simulink model "Projekt_FARE2_SS19_template_lyu"  (R2019a)
settings: Solver=ode4  StartTime=0  StopTime=5  FixedStep=0.001  MaxStep=0.001  MinStep=1e-6  RelTol=1e-3  AbsTol=1e-3
PostLoadFcn:
  | %plot(Pos_x(:,2),Pos_y(:,2));
  | %xlabel('x(m)');
  | %ylabel('y(m)');
StopFcn:
  | plot(Pos_x(:,2),Pos_y(:,2));
  | xlabel('x(m)');
  | ylabel('y(m)');
undefined symbols (not defined in the file or in its folder): in
settings Model: Creator=vivgove  LastModifiedBy=eason
settings SolverCC: AutoScaleAbsTol=off  InitialStep=0.001  MaxOrder=3  AutoInsertRateTranBlk=on  InsertRTBMode=Never (minimum delay)
settings DataIOCC: SaveFormat=Array  SignalLoggingSaveFormat=ModelDataLogs  SaveOutput=off  SignalLogging=off  SaveTime=off  ReturnWorkspaceOutputs=off  OutputOption=SpecifiedOutputTimes  OutputTimes=[time]
settings OptimizationCC: DefaultParameterBehavior=Inlined  ExpressionDepthLimit=2147483647  EfficientMapNaN2IntZero=off  LifeSpan=inf
settings DebuggingCC: UnderspecifiedInitializationDetection=Classic  MergeDetectMultiDrivingBlocksExec=none  SolverPrmCheckMsg=warning  FcnCallInpInsideContextMsg=warning  AllowSymbolicDim=off  StateNameClashWarn=warning  SFUnexpectedBacktrackingDiag=warning  SFNoUnconditionalDefaultTransitionDiag=warning  SFExecutionAtInitializationDiag=none  ArithmeticOperatorsInVariantConditions=warning
settings HardwareCC: ProdBitPerPointer=32  ProdBitPerSizeT=32  ProdBitPerPtrDiffT=32  ProdLargestAtomicFloat=None  ProdIntDivRoundTo=Undefined  ProdEndianess=Unspecified  ProdWordSize=32  ProdHWDeviceType=32-bit Generic  TargetBitPerLong=64  TargetBitPerPointer=64  TargetBitPerSizeT=64  TargetBitPerPtrDiffT=64  TargetLongLongMode=on  TargetIntDivRoundTo=Zero  TargetEndianess=LittleEndian  TargetWordSize=64  TargetHWDeviceType=MATLAB Host  ProdEqTarget=off
settings ModelReferenceCC: PropagateSignalLabelsOutOfModel=off
settings SFSimCC: SimUseLocalCustomCode=off
settings RTWCC: RTWUseLocalCustomCode=off
settings CodeAppCC: MaxIdLength=128  StateflowObjectComments=on
settings GRTTargetCC: TargetLangStandard=C89/C90 (ANSI)  CombineOutputUpdateFcns=off  GRTInterface=on
settings ConfigComp: CovMetricSettings=dw  CovHtmlReporting=on  CovSaveCumulativeToWorkspaceVar=on  CovSaveSingleToWorkspaceVar=on  CovExternalEMLEnable=off

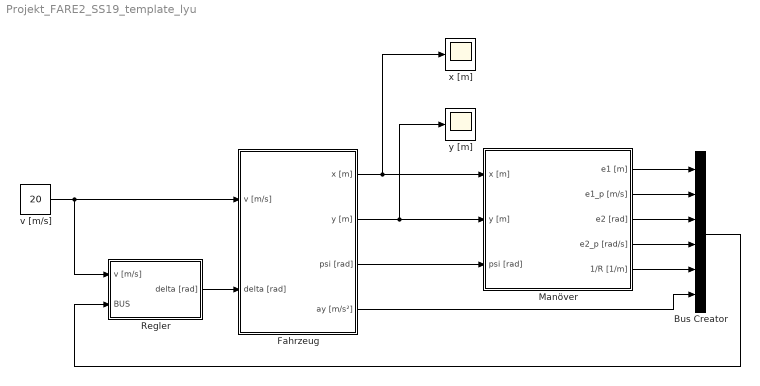
== system Projekt_FARE2_SS19_template_lyu ==
  Bus Creator : BusCreator  Inputs=6
  Fahrzeug : Subsystem
  Manöver : Subsystem
  Regler : Subsystem
  v [m/s] : Constant  Value=20
  x [m] : Scope
  y [m] : Scope
  wires:
  Manöver/1(e1 [m]) -> Bus Creator/1
  Manöver/2(e1_p [m/s]) -> Bus Creator/2
  Manöver/3(e2 [rad]) -> Bus Creator/3
  Manöver/4(e2_p [rad/s]) -> Bus Creator/4
  Manöver/5(1/R [1/m]) -> Bus Creator/5
  Bus Creator/1 -> Regler/2(BUS)
  Fahrzeug/1(x [m]) -> Manöver/1(x [m]), x [m]/1
  Fahrzeug/2(y [m]) -> Manöver/2(y [m]), y [m]/1
  Regler/1(delta [rad]) -> Fahrzeug/2(delta [rad])
  Fahrzeug/3(psi [rad]) -> Manöver/3(psi [rad])
  Fahrzeug/4(ay [m/s²]) -> Bus Creator/6
  v [m/s]/1 -> Regler/1(v [m/s]), Fahrzeug/1(v [m/s])

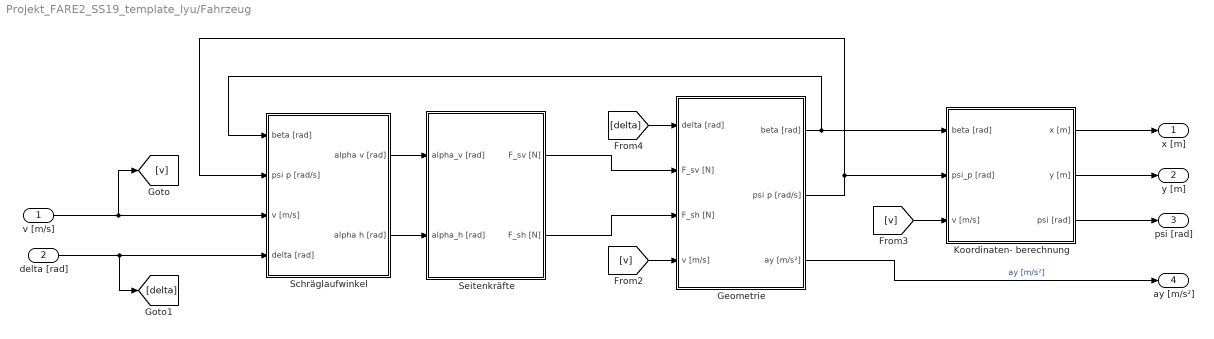
== system Projekt_FARE2_SS19_template_lyu/Fahrzeug ==
  v [m/s] : Inport
  delta [rad] : Inport  Port=2
  Geometrie : Subsystem
  Koordinaten- berechnung : Subsystem
  Schräglaufwinkel : Subsystem
  Seitenkräfte : Subsystem
  x [m] : Outport
  y [m] : Outport  Port=2
  psi [rad] : Outport  Port=3
  ay [m/s²] : Outport  Port=4
  wires:
  [v] -> Koordinaten- berechnung/3(v [m/s])
  [v] -> Geometrie/4(v [m/s])
  [delta] -> Geometrie/1(delta [rad])
  v [m/s]/1 -> Schräglaufwinkel/3(v [m/s]), [v]
  Seitenkräfte/2(F_sh [N]) -> Geometrie/3(F_sh [N])
  Koordinaten- berechnung/3(psi [rad]) -> psi [rad]/1
  Koordinaten- berechnung/1(x [m]) -> x [m]/1
  Geometrie/2(psi p [rad/s]) -> Schräglaufwinkel/2(psi p [rad/s]), Koordinaten- berechnung/2(psi_p [rad])
  Schräglaufwinkel/2(alpha h [rad]) -> Seitenkräfte/2(alpha_h [rad])
  Koordinaten- berechnung/2(y [m]) -> y [m]/1
  Seitenkräfte/1(F_sv [N]) -> Geometrie/2(F_sv [N])
  Geometrie/1(beta [rad]) -> Koordinaten- berechnung/1(beta [rad]), Schräglaufwinkel/1(beta [rad])
  Schräglaufwinkel/1(alpha v [rad]) -> Seitenkräfte/1(alpha_v [rad])
  Geometrie/3(ay [m/s²]) -> ay [m/s²]/1  "ay [m/s²]"
  delta [rad]/1 -> [delta], Schräglaufwinkel/4(delta [rad])

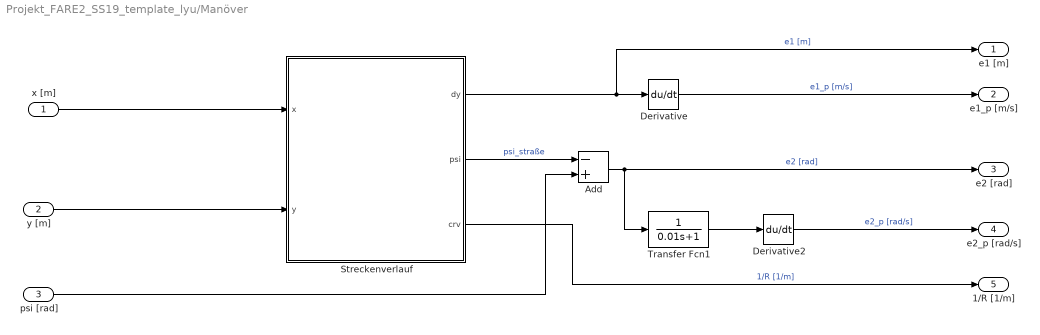
== system Projekt_FARE2_SS19_template_lyu/Manöver ==
  x [m] : Inport
  y [m] : Inport  Port=2
  psi [rad] : Inport  Port=3
  Add : Sum  Inputs=-+
  Derivative : Derivative
  Derivative2 : Derivative
  Streckenverlauf : MATLAB Function  TreatAsAtomicUnit=on
  Transfer Fcn1 : TransferFcn  Denominator=[0.01 1]
  e1 [m] : Outport
  e1_p [m/s] : Outport  Port=2
  e2 [rad] : Outport  Port=3
  e2_p [rad/s] : Outport  Port=4
  1/R [1/m] : Outport  Port=5
  wires:
  Streckenverlauf/3(crv) -> 1/R [1/m]/1  "1/R [1/m]"
  Streckenverlauf/2(psi) -> Add/1  "psi_straße"
  Streckenverlauf/1(dy) -> e1 [m]/1, Derivative/1  "e1 [m]"
  psi [rad]/1 -> Add/2
  Add/1 -> e2 [rad]/1, Transfer Fcn1/1  "e2 [rad]"
  Derivative2/1 -> e2_p [rad/s]/1  "e2_p [rad/s]"
  Transfer Fcn1/1 -> Derivative2/1
  y [m]/1 -> Streckenverlauf/2(y)
  Derivative/1 -> e1_p [m/s]/1  "e1_p [m/s]"
  x [m]/1 -> Streckenverlauf/1(x)

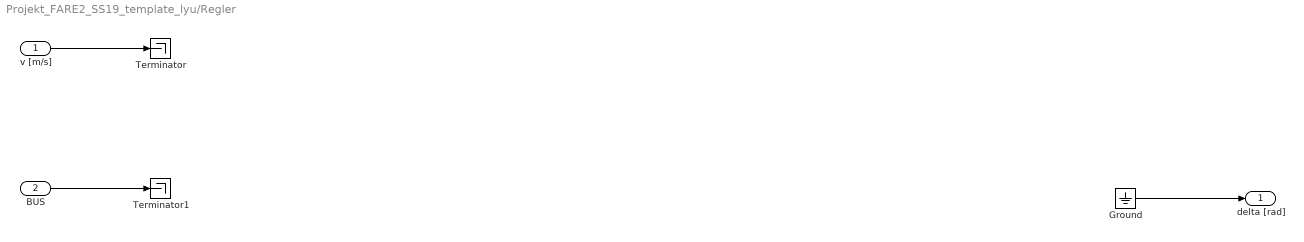
== system Projekt_FARE2_SS19_template_lyu/Regler ==
  v [m/s] : Inport
  BUS : Inport  Port=2
  Ground : Ground
  Terminator : Terminator
  Terminator1 : Terminator
  delta [rad] : Outport
  wires:
  BUS/1 -> Terminator1/1
  v [m/s]/1 -> Terminator/1
  Ground/1 -> delta [rad]/1

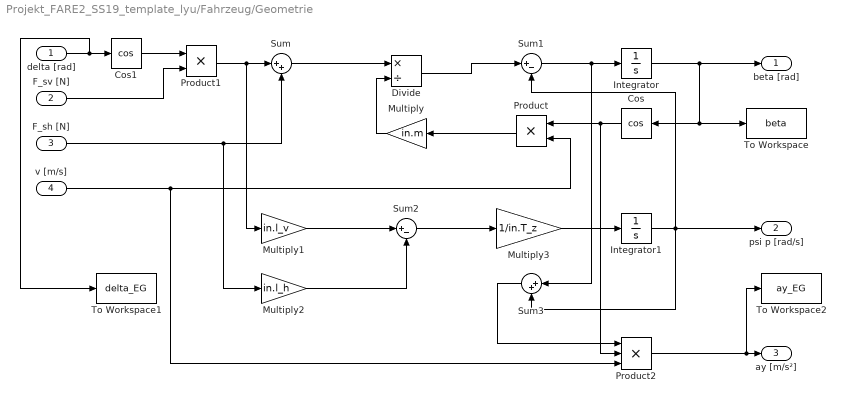
== system Projekt_FARE2_SS19_template_lyu/Fahrzeug/Geometrie ==
  delta [rad] : Inport
  F_sv [N] : Inport  Port=2
  F_sh [N] : Inport  Port=3
  v [m/s] : Inport  Port=4
  Cos : Trigonometry  Operator=cos
  Cos1 : Trigonometry  Operator=cos
  Divide : Product  Inputs=*/
  Integrator : Integrator
  Integrator1 : Integrator
  Multiply : Gain  Gain=in.m
  Multiply1 : Gain  Gain=in.l_v
  Multiply2 : Gain  Gain=in.l_h
  Multiply3 : Gain  Gain=1/in.T_z
  Product : Product
  Product1 : Product
  Product2 : Product  Inputs=3
  Sum : Sum  Inputs=|++
  Sum1 : Sum  Inputs=|+-
  Sum2 : Sum  Inputs=|+-
  Sum3 : Sum  Inputs=|++
  To Workspace : ToWorkspace  VariableName=beta  SampleTime=-1
      settings: Save2DSignal=2-D array (concatenate along first dimension)
  To Workspace1 : ToWorkspace  VariableName=delta_EG  SampleTime=-1
      settings: Save2DSignal=2-D array (concatenate along first dimension)
  To Workspace2 : ToWorkspace  VariableName=ay_EG  SampleTime=-1
      settings: Save2DSignal=2-D array (concatenate along first dimension)
  beta [rad] : Outport
  psi p [rad/s] : Outport  Port=2
  ay [m/s²] : Outport  Port=3
  wires:
  v [m/s]/1 -> Product2/3, Product/2
  Integrator/1 -> beta [rad]/1, Cos/1, To Workspace/1
  Integrator1/1 -> Sum3/2, psi p [rad/s]/1, Sum1/2
  Product2/1 -> To Workspace2/1, ay [m/s²]/1
  delta [rad]/1 -> To Workspace1/1, Cos1/1
  F_sv [N]/1 -> Product1/2
  F_sh [N]/1 -> Sum/2, Multiply2/1
  Cos/1 -> Product2/2, Product/1
  Product/1 -> Multiply/1
  Multiply/1 -> Divide/2
  Cos1/1 -> Product1/1
  Product1/1 -> Multiply1/1, Sum/1
  Sum/1 -> Divide/1
  Divide/1 -> Sum1/1
  Multiply1/1 -> Sum2/1
  Multiply2/1 -> Sum2/2
  Sum2/1 -> Multiply3/1
  Multiply3/1 -> Integrator1/1
  Sum1/1 -> Sum3/1, Integrator/1
  Sum3/1 -> Product2/1

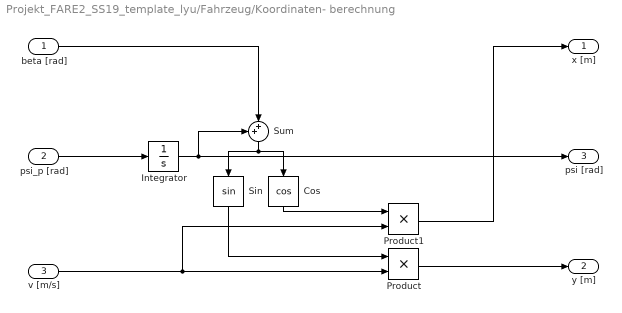
== system Projekt_FARE2_SS19_template_lyu/Fahrzeug/Koordinaten- berechnung ==
  beta [rad] : Inport
  psi_p [rad] : Inport  Port=2
  v [m/s] : Inport  Port=3
  Cos : Trigonometry  Operator=cos
  Integrator : Integrator
  Product : Product
  Product1 : Product
  Sin : Trigonometry
  Sum : Sum  Inputs=++|
  x [m] : Outport
  y [m] : Outport  Port=2
  psi [rad] : Outport  Port=3
  wires:
  psi_p [rad]/1 -> Integrator/1
  beta [rad]/1 -> Sum/2
  v [m/s]/1 -> Product/2, Product1/2
  Product1/1 -> x [m]/1
  Product/1 -> y [m]/1
  Integrator/1 -> Sum/1, psi [rad]/1
  Sum/1 -> Cos/1, Sin/1
  Sin/1 -> Product/1
  Cos/1 -> Product1/1

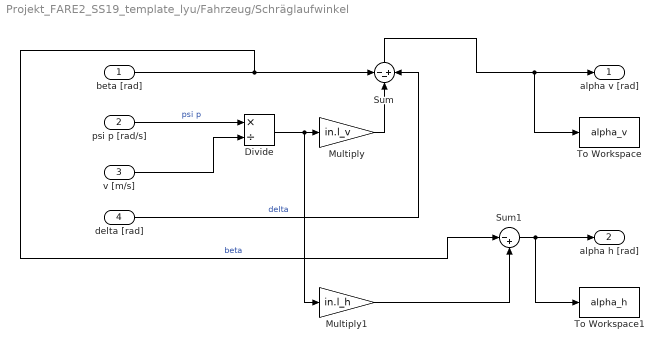
== system Projekt_FARE2_SS19_template_lyu/Fahrzeug/Schräglaufwinkel ==
  beta [rad] : Inport
  psi p [rad/s] : Inport  Port=2
  v [m/s] : Inport  Port=3
  delta [rad] : Inport  Port=4
  Divide : Product  Inputs=*/
  Multiply : Gain  Gain=in.l_v
  Multiply1 : Gain  Gain=in.l_h
  Sum : Sum  Inputs=--+
  Sum1 : Sum  Inputs=|-+
  To Workspace : ToWorkspace  VariableName=alpha_v  SampleTime=-1
      settings: Save2DSignal=2-D array (concatenate along first dimension)
  To Workspace1 : ToWorkspace  VariableName=alpha_h  SampleTime=-1
      settings: Save2DSignal=2-D array (concatenate along first dimension)
  alpha v [rad] : Outport
  alpha h [rad] : Outport  Port=2
  wires:
  beta [rad]/1 -> Sum/1, Sum1/1  "beta"
  delta [rad]/1 -> Sum/3  "delta"
  psi p [rad/s]/1 -> Divide/1  "psi p"
  Sum/1 -> To Workspace/1, alpha v [rad]/1
  Sum1/1 -> alpha h [rad]/1, To Workspace1/1
  v [m/s]/1 -> Divide/2
  Divide/1 -> Multiply1/1, Multiply/1
  Multiply/1 -> Sum/2
  Multiply1/1 -> Sum1/2

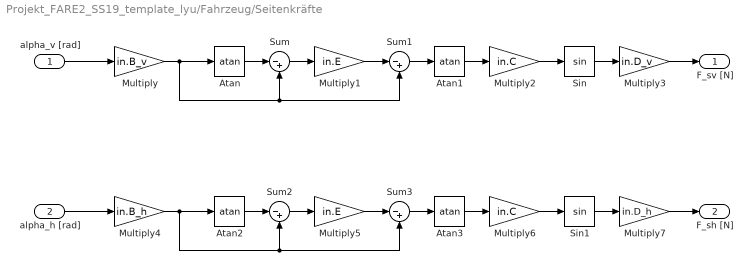
== system Projekt_FARE2_SS19_template_lyu/Fahrzeug/Seitenkräfte ==
  alpha_v [rad] : Inport
  alpha_h [rad] : Inport  Port=2
  Atan{,1..3} (4 alike) : Trigonometry  Operator=atan
  Multiply : Gain  Gain=in.B_v
  Multiply1 : Gain  Gain=in.E
  Multiply2 : Gain  Gain=in.C
  Multiply3 : Gain  Gain=in.D_v
  Multiply4 : Gain  Gain=in.B_h
  Multiply5 : Gain  Gain=in.E
  Multiply6 : Gain  Gain=in.C
  Multiply7 : Gain  Gain=in.D_h
  Sin : Trigonometry
  Sin1 : Trigonometry
  Sum{,1..3} (4 alike) : Sum  Inputs=|-+
  F_sv [N] : Outport
  F_sh [N] : Outport  Port=2
  wires:
  alpha_h [rad]/1 -> Multiply4/1
  alpha_v [rad]/1 -> Multiply/1
  Multiply3/1 -> F_sv [N]/1
  Multiply7/1 -> F_sh [N]/1
  Multiply/1 -> Sum/2, Sum1/2, Atan/1
  Atan/1 -> Sum/1
  Sum/1 -> Multiply1/1
  Multiply1/1 -> Sum1/1
  Sum1/1 -> Atan1/1
  Atan1/1 -> Multiply2/1
  Multiply2/1 -> Sin/1
  Sin/1 -> Multiply3/1
  Multiply4/1 -> Sum2/2, Sum3/2, Atan2/1
  Sum2/1 -> Multiply5/1
  Atan2/1 -> Sum2/1
  Multiply6/1 -> Sin1/1
  Sum3/1 -> Atan3/1
  Multiply5/1 -> Sum3/1
  Sin1/1 -> Multiply7/1
  Atan3/1 -> Multiply6/1

== matlab function Projekt_FARE2_SS19_template_lyu/Manöver/Streckenverlauf ==
  data: x input; data parameter; dy output; y input; psi output; crv output
function  [dy,psi,crv] = Berechnung_Streckendaten(x,data,y)
%#codegen

puv=crg_eval_xy2uv_adaptiert(data, [x y]);
psi=crg_eval_u2phi(data, puv(1));
crv=crg_eval_u2crv(data, puv(1));
dy=puv(2);
